simulink model "TV_2021"  (R2017b)
settings: Solver=VariableStepAuto  StartTime=0.0  StopTime=10.0  RelTol=1e-3
undefined symbols (not defined in the file): sigbuilder_block
libraries: simulink x6
(part 2 of 13)

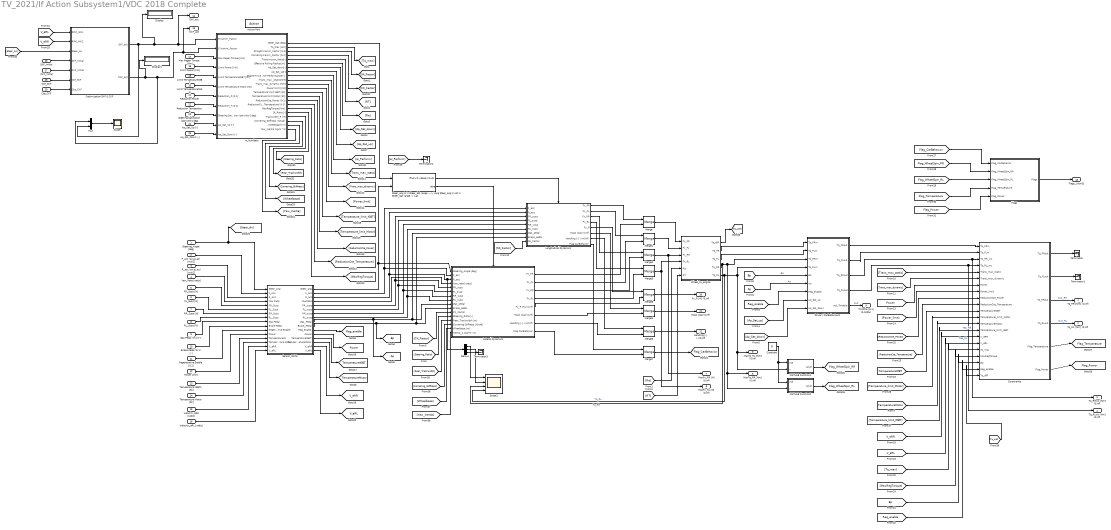
== system TV_2021/If Action Subsystem1/VDC 2018 Complete ==
  Steering_Angle [deg] : Inport
  F_acc (ax,ay,az) [m/s2] : Inport  Port=2
  R_acc (ax,ay,az) [m/s2] : Inport  Port=3
  Yaw_Rate [rad/s] : Inport  Port=4
  FR_Susp [N] : Inport  Port=5
  FL_Susp [N] : Inport  Port=6
  RR_Susp [N] : Inport  Port=7
  RL_Susp [N] : Inport  Port=8
  Gas Pedal (0-1) [-] : Inport  Port=9
  Brake Pedal (0-1) [-] : Inport  Port=10
  Regenerative Enable [0,1] : Inport  Port=11
  Power [kW] : Inport  Port=12
  Temperature IGBTs [ºC] : Inport  Port=13
  Temperature Motor [ºC] : Inport  Port=14
  Velocity_eRR [rad/s] : Inport  Port=15
  Velocity_eRL [rad/s] : Inport  Port=16
  Max Regen Torque [Nm] : Inport  Port=17
  Limit Power [kW] : Inport  Port=18
  Limit TemperatureIGBT : Inport  Port=19
  Limit TemperatureMotor : Inport  Port=20
  Reduction Power : Inport  Port=21
  Reduction Temperature : Inport  Port=22
  Steering Saturation (per site) [deg] : Inport  Port=23
  Ap_Sat_Up [-] : Inport  Port=24
  Ap_Sat_Down [-] : Inport  Port=25
  SKF_Initial : Inport  Port=26
  CKF_Initial : Inport  Port=27
  Cte_SKF : Inport  Port=28
  Cte_CKF : Inport  Port=29
  Action Port : ActionPort
  Constant : Constant  Value=0
  Constraints : Subsystem
  Demux : Demux  Outputs=3
  Display : Display
  Display1 : Display
  Driver / CarBehaviours : Subsystem
  Flags : Subsystem
  In_Numbers : Subsystem
  Lateral Dynamics : Subsystem  TreatAsAtomicUnit=on
  Longitudinal Dynamics : Subsystem  TreatAsAtomicUnit=on
  MATLAB Function1 : MATLAB Function  TreatAsAtomicUnit=on
  MATLAB Function2 : MATLAB Function  TreatAsAtomicUnit=on
  Merge{,1..7} (8 alike) : Merge
  Mux : Mux  Inputs=2
  Optimization SKF & CKF : Subsystem
  Scope : Scope
  Scope1 : Scope  NumInputPorts=4
  Sensor_DATA : Subsystem
  "Steer_ang is in Steer_Sat range ---> Long Steer_ang is not in Steer_Sat range -> Lat " : If  NumInputs=2  IfExpression=u2>=-u1&u2<=u1
  Terminator{,1..3} (4 alike) : Terminator
  Wheel_to_engine : Subsystem
  Tq_RR [Nm] (0,inf) : Outport
  Tq_RL [Nm] (0,inf) : Outport  Port=2
  Tq_RRwc [Nm] (0,inf) : Outport  Port=3
  Tq_RLwc [Nm] (0,inf) : Outport  Port=4
  MaxTq_RR [Nm] (0,inf) : Outport  Port=5
  MaxTq_RL [Nm] (0,inf) : Outport  Port=6
  MaxFx_RR [N] (0,inf) : Outport  Port=7
  MaxFx_RL [N] (0,inf) : Outport  Port=8
  Throttle [0-1] (0-100%) : Outport  Port=9
  Fy_R [N] (0,inf) : Outport  Port=10
  Mass [kg] (0,inf) : Outport  Port=11
  Handling [-] (-inf,inf) : Outport  Port=12
  Flags_[num5] : Outport  Port=13
  SKF_act : Outport  Port=14
  CKF_act : Outport  Port=15
  tag scope: Ap=global, Bp=global, Flag_CarBehavior=global, Flag_Power=global, Flag_Temperature=global, Flag_WheelSpin_RL=global, Flag_WheelSpin_RR=global, Power=global, Reg_enable=global, TemperatureIGBT=global, TemperatureMotor=global, V_eRL=global, V_eRR=global
  wires:
  "Steer_ang is in Steer_Sat range ---> Long Steer_ang is not in Steer_Sat range -> Lat "/1 -> Longitudinal Dynamics/Action
  "Steer_ang is in Steer_Sat range ---> Long Steer_ang is not in Steer_Sat range -> Lat "/2 -> Lateral Dynamics/Action
  Sensor_DATA/8(RL_susp) -> Longitudinal Dynamics/6(RL_susp), Lateral Dynamics/8(RL_susp)
  In_Numbers/3(Straight Kamm_Factor [0-2]) -> [SK_Factor]
  In_Numbers/1(Steer_Sat [deg]) -> "Steer_ang is in Steer_Sat range ---> Long Steer_ang is not in Steer_Sat range -> Lat "/1
  In_Numbers/2(Tq_Max [Nm]) -> [Tq_max]
  Sensor_DATA/9(Gas_Pedal) -> [Ap], Lateral Dynamics/9(Gas_pedal), Longitudinal Dynamics/7(Gas_pedal)
  In_Numbers/6(Effective Rolling Radius[m]) -> [Re]
  In_Numbers/5(Transmision_Ratio[-]) -> [RT]
  Sensor_DATA/7(RR_susp) -> Longitudinal Dynamics/5(RR_susp), Lateral Dynamics/7(RR_susp)
  In_Numbers/8(Ap_Sat_up[-]) -> [Ap_Sat_up]
  In_Numbers/7(Ap_Sat_down[-]) -> [Ap_Sat_down]
  Driver / CarBehaviours/3(Tq_RRout) -> Tq_RRwc [Nm] (0,inf)/1, Constraints/3(Tq_RR_wc)  "Teo_RR"
  Sensor_DATA/2(F_acc) -> Longitudinal Dynamics/1(F_acc), Lateral Dynamics/2(F_acc)
  Sensor_DATA/3(R_acc) -> Longitudinal Dynamics/2(R_acc), Demux/1, Lateral Dynamics/3(R_acc)
  Sensor_DATA/10(Brake_Pedal) -> [Bp], Lateral Dynamics/10(Brake_pedal), Longitudinal Dynamics/8(Brake_pedal)
  Sensor_DATA/6(FL_susp) -> Longitudinal Dynamics/4(FL_susp), Lateral Dynamics/6(FL_susp)
  Sensor_DATA/11(Reg_Enable) -> [Reg_enable]
  Sensor_DATA/5(FR_susp) -> Longitudinal Dynamics/3(FR_susp), Lateral Dynamics/5(FR_susp)
  Sensor_DATA/1(Steer_ang) -> Lateral Dynamics/1(Steering_Angle [deg]), "Steer_ang is in Steer_Sat range ---> Long Steer_ang is not in Steer_Sat range -> Lat "/2
  Wheel_to_engine/5(Tq_RL) -> Scope1/4, MaxTq_RL [Nm] (0,inf)/1, MATLAB Function1/2(v), Driver / CarBehaviours/4("Tq_RLin ")  "Tq_RL"
  [Trans_max_dynamic] -> Constraints/6(Trans_max_dynamic)
  [Power_limit] -> Constraints/8(Power_limit)
  In_Numbers/15(ReductionCte_Power (0-1)) -> [ReductionCte_Power]
  Driver / CarBehaviours/5(out_Throttle) -> Throttle [0-1] (0-100%)/1  "Out"
  Wheel_to_engine/4(Tq_RR) -> Scope1/3, MATLAB Function2/2(v), MaxTq_RR [Nm] (0,inf)/1, Driver / CarBehaviours/3(Tq_RRin)  "Tq_RR"
  Wheel_to_engine/3(Tq_FL) -> Driver / CarBehaviours/2(Tq_FLin)
  In_Numbers/11(Trans_max_dynamic [Nm]) -> [Trans_max_dynamic]
  [Reg_enable] -> Driver / CarBehaviours/7(Reg_enable)
  [ReductionCte_Power] -> Constraints/9(ReductionCte_Power)
  [Ap_Sat_up] -> Driver / CarBehaviours/8(Ap_Sat_up)
  In_Numbers/10(Trans_max _static[Nm]) -> [Trans_max_static]
  [Ap] -> Driver / CarBehaviours/6(Ap)  "Ap"
  [Power] -> Constraints/7(Power)
  In_Numbers/12("Power limit [KW] ") -> [Power_limit]
  [Ap_Sat_down] -> Driver / CarBehaviours/9(Ap_Sat_down)
  Driver / CarBehaviours/4(Tq_RLout) -> Tq_RLwc [Nm] (0,inf)/1, Constraints/4("Tq_RL_wc ")  "Teo_RL"
  Driver / CarBehaviours/2("Tq_FLout ") -> Constraints/2(Tq_FLin)
  Steering_Angle [deg]/1 -> [Steer_An], Sensor_DATA/1(Steer_Ang)
  Wheel_to_engine/2(Tq_FR) -> Driver / CarBehaviours/1(Tq_FRin)
  Driver / CarBehaviours/1(Tq_FRout) -> Constraints/1(Tq_FRin)
  [Trans_max_static] -> Constraints/5("Trans_max_static ")
  [Temperature_limit_IGBT] -> Constraints/14(Temperature_limit_IGBT)
  [Bp] -> Constraints/19(Bp)
  Sensor_DATA/16(V_eRL) -> [V_eRL]
  In_Numbers/17(MaxRegTorque [Nm]) -> [MaxRegTorque]
  [TemperatureIGBT] -> Constraints/11(TemperatureIGBT)
  [Reg_enable] -> Constraints/20(Reg_enable)
  In_Numbers/9(Engine+Inverter Performance[-]) -> [ei_Perform]
  [Bp] -> Driver / CarBehaviours/5(Bp)  "Bp"
  [Tq_max] -> Constraints/17(Tq_max)
  RR_Susp [N]/1 -> Sensor_DATA/7(RR_Susp)
  Power [kW]/1 -> Sensor_DATA/12("Power ")
  Sensor_DATA/12(Power) -> [Power]
  Sensor_DATA/15("V_eRR ") -> [V_eRR]
  [V_eRR] -> Constraints/15(V_eRR)
  Regenerative Enable [0,1]/1 -> Sensor_DATA/11(Regenerative Enable)
  Brake Pedal (0-1) [-]/1 -> Sensor_DATA/10(Brake Pedal)
  [V_eRL] -> Constraints/16(V_eRL)
  In_Numbers/13(Temperature limit IGBT [ºC]) -> [Temperature_limit_IGBT]
  FL_Susp [N]/1 -> Sensor_DATA/6(FL_Susp)
  FR_Susp [N]/1 -> Sensor_DATA/5(FR_Susp)
  R_acc (ax,ay,az) [m/s2]/1 -> Sensor_DATA/3(R_Acc)
  F_acc (ax,ay,az) [m/s2]/1 -> Sensor_DATA/2("F_Acc ")
  RL_Susp [N]/1 -> Sensor_DATA/8(RL_Susp)
  Gas Pedal (0-1) [-]/1 -> Sensor_DATA/9(Gas Pedal)
  Temperature IGBTs [ºC]/1 -> Sensor_DATA/13(TemperatureIN)
  Velocity_eRR [rad/s]/1 -> Sensor_DATA/15(V_eRR)
  Velocity_eRL [rad/s]/1 -> Sensor_DATA/16("V_eRL ")
  Constraints/1(Tq_FRout) -> Terminator/1
  Constraints/2("Tq_FLout ") -> Terminator1/1
  In_Numbers/4(Cornering Kamm_Factor [0-2]) -> [CK_Factor]
  [Re] -> Wheel_to_engine/5(Re)
  [RT] -> Wheel_to_engine/6(RT)
  Merge3/1 -> MaxFx_RL [N] (0,inf)/1, Wheel_to_engine/4("Fx_RL ")
  Merge2/1 -> Wheel_to_engine/3("Fx_RR "), MaxFx_RR [N] (0,inf)/1
  Merge1/1 -> Wheel_to_engine/2("Fx_FL ")
  Max Regen Torque [Nm]/1 -> In_Numbers/3(Max Regen Torque [Nm])
  Limit Power [kW]/1 -> In_Numbers/4(Limit Power [kW])
  Limit TemperatureIGBT/1 -> In_Numbers/5(Limit TemperatureIGBT [ºC])
  Reduction Power/1 -> In_Numbers/7(Reduction_P [0-1])
  [CK_Factor] -> Lateral Dynamics/11(CK_Factor)
  [SK_Factor] -> Longitudinal Dynamics/9(SK_Factor)
  Longitudinal Dynamics/1(Fx_FR) -> Merge/1
  Longitudinal Dynamics/2(Fx_FL) -> Merge1/1
  Longitudinal Dynamics/3("Fx_RR ") -> Merge2/1
  Longitudinal Dynamics/4("Fx_RL ") -> Merge3/1
  Lateral Dynamics/1(Fx_FR) -> Merge/2
  Lateral Dynamics/2(Fx_FL) -> Merge1/2
  Lateral Dynamics/3("Fx_RR ") -> Merge2/2
  Lateral Dynamics/4("Fx_RL ") -> Merge3/2
  Merge/1 -> Wheel_to_engine/1("Fx_FR ")
  Steering Saturation (per site) [deg]/1 -> In_Numbers/9(Steering Saturation (per site) [deg])
  Ap_Sat_Up [-]/1 -> In_Numbers/10(Ap_Sat_Up [-])
  Ap_Sat_Down [-]/1 -> In_Numbers/11(Ap_Sat_Down [-])
  [MaxRegTorque] -> Constraints/18(MaxRegTorque)
  [ei_Perform] -> Terminator2/1
  Merge4/1 -> Mass [kg] (0,inf)/1
  Longitudinal Dynamics/6(Mass [kg] (0,inf)) -> Merge4/1
  Lateral Dynamics/6(" Mass [kg] (0,inf)") -> Merge4/2
  Longitudinal Dynamics/7(Handling [-] (-inf,inf)) -> Merge5/1
  Lateral Dynamics/7(Handling [-] (-inf,inf)) -> Merge5/2
  Merge5/1 -> Handling [-] (-inf,inf)/1
  Merge6/1 -> Fy_R [N] (0,inf)/1
  Lateral Dynamics/5(Fy_R [N] (0,inf)) -> Merge6/2
  Longitudinal Dynamics/5(Fy_R) -> Merge6/1
  In_Numbers/16(ReductionCte_Temperature (0-1)) -> [ReductionCte_Temperature]
  Reduction Temperature/1 -> In_Numbers/8(Reduction_T [0-1])
  [ReductionCte_Temperature] -> Constraints/10(ReductionCte_Temperature)
  Constraints/3(Tq_RRout) -> Tq_RR [Nm] (0,inf)/1  "Out_RR"
  Constraints/4(Tq_RLout) -> Tq_RL [Nm] (0,inf)/1  "Out_RL"
  Temperature Motor [ºC]/1 -> Sensor_DATA/14(Temperature Motor)
  Sensor_DATA/13(TemperatureIGBT) -> [TemperatureIGBT]
  Sensor_DATA/14(TemperatureMotor) -> [TemperatureMotor]
  [TemperatureMotor] -> Constraints/13(TemperatureIMotor)
  [Temperature_limit_Motor] -> Constraints/12(TemperatureI_limit_Motor)
  In_Numbers/14(Temperature limit Motor [ºC]) -> [Temperature_limit_Motor]
  Limit TemperatureMotor/1 -> In_Numbers/6(Limit Temperature Motor [ºC])
  Merge7/1 -> [Flag_CarBehavior]
  Longitudinal Dynamics/8(Flag CarBehavior) -> Merge7/1
  Lateral Dynamics/8(Flag CarBehavior) -> Merge7/2
  MATLAB Function2/1(value) -> [Flag_WheelSpin_RL]
  MATLAB Function1/1(value) -> [Flag_WheelSpin_RR]
  Constant/1 -> MATLAB Function2/1(cte), MATLAB Function1/1(cte)
  Constraints/5(Flag_Temperature) -> [Flag_Temperature]
  Constraints/6(Flag_Power) -> [Flag_Power]
  Flags/1(Flags) -> Flags_[num5]/1
  [Flag_WheelSpin_RL] -> Flags/3(Flag_WheelSpin_RL)
  [Flag_WheelSpin_RR] -> Flags/2(Flag_WheelSpin_RR)
  [Flag_CarBehavior] -> Flags/1(Flag_CarBehavior)
  [Flag_Temperature] -> Flags/4(Flag_Temperature)
  [Flag_Power] -> Flags/5(Flag_Power)
  Optimization SKF & CKF/1(SKF_act) -> In_Numbers/1(S-Kamm_Factor), SKF_act/1, Display/1, Mux/2
  CKF_Initial/1 -> Optimization SKF & CKF/5(CKF_Initial)
  [Steer_An] -> Optimization SKF & CKF/3(Steer_An)
  [V_eRR] -> Optimization SKF & CKF/2(RPM_INV2)
  Cte_SKF/1 -> Optimization SKF & CKF/6(Cte_SKF)
  Cte_CKF/1 -> Optimization SKF & CKF/7(Cte_CKF)
  SKF_Initial/1 -> Optimization SKF & CKF/4(SKF_Initial)
  [V_eRL] -> Optimization SKF & CKF/1(RPM_INV1)
  Optimization SKF & CKF/2(CKF_act) -> Display1/1, Mux/1, In_Numbers/2(C-Kamm_Factor), CKF_act/1
  Mux/1 -> Scope/1
  Yaw_Rate [rad/s]/1 -> Sensor_DATA/4(Yaw Rate)
  Sensor_DATA/4(YawRate) -> Lateral Dynamics/4(Yaw_rate [rad/s])
  In_Numbers/18(St_Ratio [-]) -> [Steering_Ratio]
  [Steering_Ratio] -> Lateral Dynamics/12(Steering_Ratio [-])
  Demux/2 -> Scope1/2
  Demux/1 -> Scope1/1
  Demux/3 -> Terminator3/1
  In_Numbers/19(Trackwidth_R (m)) -> [Rear_Trackwidth]
  In_Numbers/20(Cornering_Stiffness (N/rad)) -> [Cornering_Stiffness]
  In_Numbers/21(Wheelbase (m)) -> [Wheelbase]
  [Rear_Trackwidth] -> Lateral Dynamics/13(Rear_Trackwidth [m])
  [Cornering_Stiffness] -> Lateral Dynamics/14(Cornering Stiffness [N/rad])
  [Wheelbase] -> Lateral Dynamics/15(Wheelbase [m])
  In_Numbers/22(Yaw_Inertia (kg/m^3)) -> [Yaw_Inertia]
  [Yaw_Inertia] -> Lateral Dynamics/16(Inertia_Z [kg*m^2])
  Wheel_to_engine/1(Tq_diff) -> [Tq_diff]
  [Tq_diff] -> Constraints/21(Tq_diff)

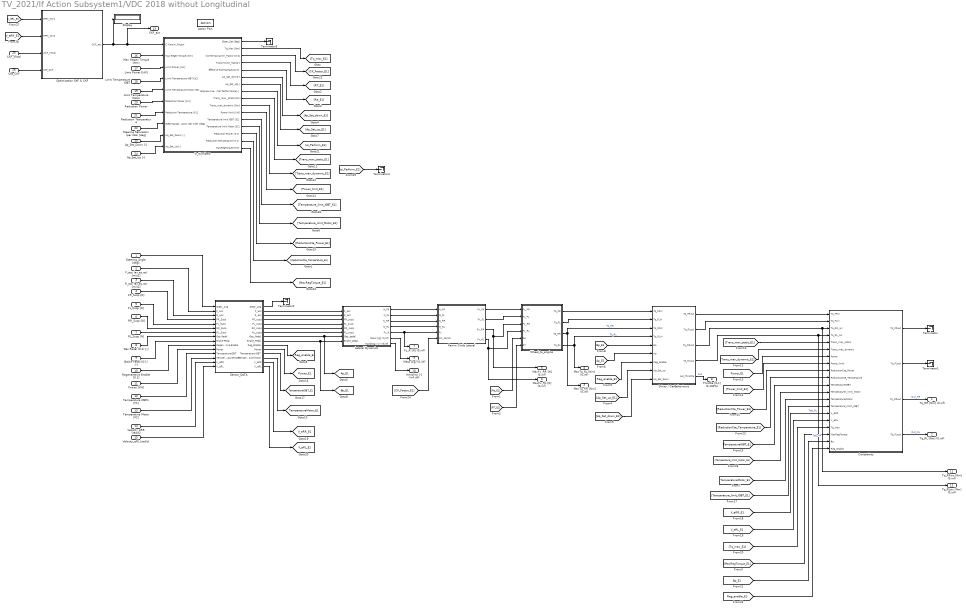
== system TV_2021/If Action Subsystem1/VDC 2018 without Longitudinal ==
  Steering_Angle [deg] : Inport
  F_acc (ax,ay,az) [m/s2] : Inport  Port=2
  R_acc (ax,ay,az) [m/s2] : Inport  Port=3
  FR_Susp [N] : Inport  Port=4
  FL_Susp [N] : Inport  Port=5
  RR_Susp [N] : Inport  Port=6
  RL_Susp [N] : Inport  Port=7
  Gas Pedal (0-1) [-] : Inport  Port=8
  Brake Pedal (0-1) [-] : Inport  Port=9
  Regenerative Enable [0,1] : Inport  Port=10
  Power [kW] : Inport  Port=11
  Temperature IGBTs [ºC] : Inport  Port=12
  Temperature Motor [ºC] : Inport  Port=13
  Velocity_eRR [rad/s] : Inport  Port=14
  Velocity_eRL [rad/s] : Inport  Port=15
  Max Regen Torque [Nm] : Inport  Port=16
  Limit Power [kW] : Inport  Port=17
  Limit Temperature IGBT : Inport  Port=18
  Limit Temperature Motor : Inport  Port=19
  Reduction Power : Inport  Port=20
  Reduction Temperature : Inport  Port=21
  Steering Saturation (per site) [deg] : Inport  Port=22
  Ap_Sat_Down [-] : Inport  Port=23
  Ap_Sat_Up [-] : Inport  Port=24
  CKF_Initial : Inport  Port=25
  Cte_CKF : Inport  Port=26
  Action Port : ActionPort
  Constraints : Subsystem
  Display : Display
  Driver / CarBehaviours : Subsystem
  In_Numbers : Subsystem
  Kamm Circle Lateral : Subsystem
  Lateral Dynamics : Subsystem
  Optimization SKF & CKF : Subsystem
  Sensor_DATA : Subsystem
  Terminator{,1..2,4..5} (5 alike) : Terminator
  Wheel_to_engine : Subsystem
  Tq_RR [Nm] (0,inf) : Outport
  Tq_RL [Nm] (0,inf) : Outport  Port=2
  MaxTq_RR [Nm] (0,inf) : Outport  Port=3
  MaxTq_RL [Nm] (0,inf) : Outport  Port=4
  MaxFx_RR [N] (0,inf) : Outport  Port=5
  MaxFx_RL [N] (0,inf) : Outport  Port=6
  Fy_R [N] (0,inf) : Outport  Port=7
  Throttle [0-1] (0-100%) : Outport  Port=8
  Mass [kg] (0,inf) : Outport  Port=9
  Handling [-] (-inf,inf) : Outport  Port=10
  Tq_RRwc [Nm] (0,inf) : Outport  Port=11
  Tq_RLwc [Nm] (0,inf) : Outport  Port=12
  CKF_act : Outport  Port=13
  tag scope: Ap_E1=global, Bp_E1=global, Power_E1=global, Reg_enable_E1=global, TemperatureIGBT_E1=global, TemperatureMotor_E1=global, V_eRL_E1=global, V_eRR_E1=global
  wires:
  Sensor_DATA/7(RL_susp) -> Lateral Dynamics/6(RL_susp)
  In_Numbers/2(Tq_Max [Nm]) -> [Tq_max_E1]
  Sensor_DATA/8(Gas_Pedal) -> [Ap_E1], Lateral Dynamics/7(Gas_pedal)
  In_Numbers/5(Effective Rolling Radius[m]) -> [Re_E1]
  In_Numbers/4(Transmision_Ratio[-]) -> [RT_E1]
  Sensor_DATA/6(RR_susp) -> Lateral Dynamics/5(RR_susp)
  In_Numbers/7(Ap_Sat_up[-]) -> [Ap_Sat_up_E1]
  In_Numbers/6(Ap_Sat_down[-]) -> [Ap_Sat_down_E1]
  Sensor_DATA/2(F_acc) -> Lateral Dynamics/1(F_acc)
  Sensor_DATA/3(R_acc) -> Lateral Dynamics/2(R_acc)
  Sensor_DATA/9(Brake_Pedal) -> [Bp_E1], Lateral Dynamics/8(Brake_pedal)
  Sensor_DATA/5(FL_susp) -> Lateral Dynamics/4(FL_susp)
  Sensor_DATA/10(Reg_Enable) -> [Reg_enable_E1]
  Sensor_DATA/4(FR_susp) -> Lateral Dynamics/3(FR_susp)
  Wheel_to_engine/4(Tq_RL) -> MaxTq_RL [Nm] (0,inf)/1, Driver / CarBehaviours/4("Tq_RLin ")  "Tq_RL"
  In_Numbers/14(Reduction Power (0-1)) -> [ReductionCte_Power_E1]
  Wheel_to_engine/3(Tq_RR) -> MaxTq_RR [Nm] (0,inf)/1, Driver / CarBehaviours/3(Tq_RRin)  "Tq_RR"
  Wheel_to_engine/2(Tq_FL) -> Driver / CarBehaviours/2(Tq_FLin)
  In_Numbers/10(Trans_max_dynamic [Nm]) -> [Trans_max_dynamic_E1]
  [Reg_enable_E1] -> Driver / CarBehaviours/7(Reg_enable)
  [Ap_Sat_up_E1] -> Driver / CarBehaviours/8(Ap_Sat_up)
  In_Numbers/9(Trans_max _static[Nm]) -> [Trans_max_static_E1]
  [Ap_E1] -> Driver / CarBehaviours/6(Ap)
  In_Numbers/11("Power limit [KW] ") -> [Power_limit_E1]
  [Ap_Sat_down_E1] -> Driver / CarBehaviours/9(Ap_Sat_down)
  Steering_Angle [deg]/1 -> Sensor_DATA/1(Steer_Ang)
  Wheel_to_engine/1(Tq_FR) -> Driver / CarBehaviours/1(Tq_FRin)
  Sensor_DATA/15(V_eRL) -> [V_eRL_E1]
  In_Numbers/16(MaxRegTorque [Nm]) -> [MaxRegTorque_E1]
  In_Numbers/8(Engine+Inverter Performance[-]) -> [ei_Perform_E1]
  [Bp_E1] -> Driver / CarBehaviours/5(Bp)
  Sensor_DATA/12(Temperature IGBT) -> [TemperatureIGBT_E1]
  RR_Susp [N]/1 -> Sensor_DATA/6(RR_Susp)
  Power [kW]/1 -> Sensor_DATA/11("Power ")
  Sensor_DATA/11(Power) -> [Power_E1]
  Sensor_DATA/14("V_eRR ") -> [V_eRR_E1]
  Regenerative Enable [0,1]/1 -> Sensor_DATA/10(Regenerative Enable)
  Brake Pedal (0-1) [-]/1 -> Sensor_DATA/9(Brake Pedal)
  In_Numbers/12(Temperature limit IGBT [ºC]) -> [Temperature_limit_IGBT_E1]
  FL_Susp [N]/1 -> Sensor_DATA/5(FL_Susp)
  FR_Susp [N]/1 -> Sensor_DATA/4(FR_Susp)
  R_acc (ax,ay,az) [m/s2]/1 -> Sensor_DATA/3(R_Acc)
  F_acc (ax,ay,az) [m/s2]/1 -> Sensor_DATA/2("F_Acc ")
  RL_Susp [N]/1 -> Sensor_DATA/7(RL_Susp)
  Gas Pedal (0-1) [-]/1 -> Sensor_DATA/8(Gas Pedal)
  Temperature IGBTs [ºC]/1 -> Sensor_DATA/12(TemperatureIGBT)
  Velocity_eRR [rad/s]/1 -> Sensor_DATA/14(V_eRR)
  Velocity_eRL [rad/s]/1 -> Sensor_DATA/15("V_eRL ")
  Max Regen Torque [Nm]/1 -> In_Numbers/2(Max Regen Torque [Nm])
  Limit Power [kW]/1 -> In_Numbers/3(Limit Power [kW])
  Limit Temperature IGBT/1 -> In_Numbers/4(Limit Temperature IGBT [ºC])
  Reduction Power/1 -> In_Numbers/6(Reduction Power [0-1])
  In_Numbers/3(Cornering Kamm_Factor [0-2]) -> [CK_Factor_E1]
  [Re_E1] -> Wheel_to_engine/5(Re)
  [RT_E1] -> Wheel_to_engine/6(RT)
  Ap_Sat_Up [-]/1 -> In_Numbers/10(Ap_Sat_Up [-])
  Ap_Sat_Down [-]/1 -> In_Numbers/9(Ap_Sat_Down [-])
  Steering Saturation (per site) [deg]/1 -> In_Numbers/8(Steering Saturation (per site) [deg])
  [CK_Factor_E1] -> Kamm Circle Lateral/6(CK_Factor)
  Kamm Circle Lateral/1(Fx_FR) -> Wheel_to_engine/1("Fx_FR ")
  Kamm Circle Lateral/2(Fx_FL) -> Wheel_to_engine/2("Fx_FL ")
  Kamm Circle Lateral/3("Fx_RR ") -> MaxFx_RR [N] (0,inf)/1, Wheel_to_engine/3("Fx_RR ")
  Kamm Circle Lateral/4("Fx_RL ") -> MaxFx_RL [N] (0,inf)/1, Wheel_to_engine/4("Fx_RL ")
  Sensor_DATA/1(Steer_ang) -> Terminator2/1
  Lateral Dynamics/1(N_FR) -> Kamm Circle Lateral/1("N_FR ")
  Lateral Dynamics/2("N_FL ") -> Kamm Circle Lateral/2(N_FL)
  Lateral Dynamics/3("N_RR ") -> Kamm Circle Lateral/3(N_RR)
  Lateral Dynamics/4(N_RL) -> Kamm Circle Lateral/4(N_RL)
  Lateral Dynamics/5(Fy_R) -> Fy_R [N] (0,inf)/1, Kamm Circle Lateral/5(Fy)
  Driver / CarBehaviours/5(out_Throttle) -> Throttle [0-1] (0-100%)/1  "Out"
  [ei_Perform_E1] -> Terminator4/1
  In_Numbers/1(Steer_Sat [deg]) -> Terminator5/1
  Lateral Dynamics/6(Mass [kg] (0,inf)) -> Mass [kg] (0,inf)/1
  Lateral Dynamics/7(Handling [-] (-inf,inf)) -> Handling [-] (-inf,inf)/1
  In_Numbers/15(Reduction Temperature (0-1)) -> [ReductionCte_Temperature_E1]
  Reduction Temperature/1 -> In_Numbers/7(Reduction Temperature [0-1])
  Driver / CarBehaviours/3(Tq_RRout) -> Tq_RRwc [Nm] (0,inf)/1, Constraints/3(Tq_RR_wc)  "Teo_RR"
  [Trans_max_dynamic_E1] -> Constraints/6(Trans_max_dynamic)
  [Power_limit_E1] -> Constraints/8(Power_limit)
  [ReductionCte_Power_E1] -> Constraints/9(ReductionCte_Power)
  [Power_E1] -> Constraints/7(Power)
  Driver / CarBehaviours/4(Tq_RLout) -> Tq_RLwc [Nm] (0,inf)/1, Constraints/4("Tq_RL_wc ")  "Teo_RL"
  Driver / CarBehaviours/2("Tq_FLout ") -> Constraints/2(Tq_FLin)
  Driver / CarBehaviours/1(Tq_FRout) -> Constraints/1(Tq_FRin)
  [Trans_max_static_E1] -> Constraints/5("Trans_max_static ")
  [Temperature_limit_IGBT_E1] -> Constraints/14(Temperature_limit_IGBT)
  [Bp_E1] -> Constraints/19(Bp)
  [TemperatureIGBT_E1] -> Constraints/11(TemperatureIGBT)
  [Reg_enable_E1] -> Constraints/20(Reg_enable)
  [Tq_max_E1] -> Constraints/17(Tq_max)
  [V_eRR_E1] -> Constraints/15(V_eRR)
  [V_eRL_E1] -> Constraints/16(V_eRL)
  Constraints/1(Tq_FRout) -> Terminator/1
  Constraints/2("Tq_FLout ") -> Terminator1/1
  [MaxRegTorque_E1] -> Constraints/18(MaxRegTorque)
  [ReductionCte_Temperature_E1] -> Constraints/10(ReductionCte_Temperature)
  Constraints/3(Tq_RRout) -> Tq_RR [Nm] (0,inf)/1  "Out_RR"
  Constraints/4(Tq_RLout) -> Tq_RL [Nm] (0,inf)/1  "Out_RL"
  [TemperatureMotor_E1] -> Constraints/13(TemperatureIMotor)
  [Temperature_limit_Motor_E1] -> Constraints/12(TemperatureI_limit_Motor)
  Limit Temperature Motor/1 -> In_Numbers/5(Limit Temperature Motor [ºC])
  In_Numbers/13(Temperature limit Motor [ºC]) -> [Temperature_limit_Motor_E1]
  Temperature Motor [ºC]/1 -> Sensor_DATA/13(TemperatureMotor)
  Sensor_DATA/13(Temperature Motor) -> [TemperatureMotor_E1]
  [V_eRR_E1] -> Optimization SKF & CKF/2(RPM_INV2)
  CKF_Initial/1 -> Optimization SKF & CKF/3(CKF_Initial)
  Cte_CKF/1 -> Optimization SKF & CKF/4(Cte_CKF)
  Optimization SKF & CKF/1(CKF_act) -> Display/1, In_Numbers/1(C-Kamm_Factor), CKF_act/1
  [V_eRL_E1] -> Optimization SKF & CKF/1(RPM_INV1)

== system TV_2021/Vehicle Dynamics Control 1/Rigid Axle ==
  "Ap_Sat_up " : Inport
  Ap_Sat_down : Inport  Port=2
  Gas Pedal [0-1] : Inport  Port=3
  Action Port : ActionPort
  Accelerating : Subsystem
  Torque_RL [Nm] : Constant  Value=60
  Torque_RR [Nm] : Constant  Value=60
  Tq_RR_E3 : Outport
  Tq_RL_E3 : Outport  Port=2
  wires:
  Ap_Sat_down/1 -> Accelerating/3(Ap_Sat_down)
  "Ap_Sat_up "/1 -> Accelerating/2("Ap_Sat_up ")
  Gas Pedal [0-1]/1 -> Accelerating/1(Ap)
  Accelerating/1("Tq_RR ") -> Tq_RR_E3/1
  Accelerating/2(Tq_RL) -> Tq_RL_E3/1
  Torque_RL [Nm]/1 -> Accelerating/5("Tq_RL ")
  Torque_RR [Nm]/1 -> Accelerating/4(Tq_RR)

== system TV_2021/Vehicle Dynamics Control 1/Steering TV 2017 with TC ==
  "Ap_Sat_up " : Inport
  Ap_Sat_down : Inport  Port=2
  Gas Pedal [0-1] : Inport  Port=3
  Steering_Angle [deg] : Inport  Port=4
  "Steering Wheel Saturation (per site) " : Inport  Port=5
  Power : Inport  Port=6
  Temperature_limit_IGBT : Inport  Port=7
  TemperatureIGBT : Inport  Port=8
  Temperature_limit_Motor : Inport  Port=9
  TemperatureMotor : Inport  Port=10
  Reduction_Power : Inport  Port=11
  Reduction_Temperature : Inport  Port=12
  SKF_Initial : Inport  Port=13
  CKF_Initial : Inport  Port=14
  Cte_SKF : Inport  Port=15
  Cte_CKF : Inport  Port=16
  Vel_eRL : Inport  Port=17
  Vel_eRR : Inport  Port=18
  Temp_Celdas : Inport  Port=19
  Lim_Temp_Celdas : Inport  Port=20
  Voltage : Inport  Port=21
  Corriente : Inport  Port=22
  Action Port : ActionPort
  Accelerating : Subsystem
  CKF : Display
  Constraints : Subsystem
  Display{2..6} (5 alike) : Display
  If : If  NumInputs=2  IfExpression=-u2 <= u1 & u1 <= u2
  Lateral Dynamics : Subsystem  TreatAsAtomicUnit=on
  Longitudinal Dynamics : Subsystem  TreatAsAtomicUnit=on
  MATLAB Function1 : MATLAB Function  TreatAsAtomicUnit=on
  Merge : Merge
  Merge1 : Merge
  Mux : Mux  Inputs=2
  Optimization SKF & CKF : Subsystem
  SKF : Display
  Scope : Scope
  Steering TV 2017 without TC : MATLAB Function  TreatAsAtomicUnit=on
  Steering Wheel Maximum Angle : Constant  Value=140
  Tq_diff_max [Nm] : Constant  Value=100
  Tq_max [Nm] : Constant  Value=130
  Tq_RR_E2 : Outport
  Tq_RL_E2 : Outport  Port=2
  SKF_act : Outport  Port=3
  CKF_act : Outport  Port=4
  wires:
  Corriente/1 -> Constraints/13(Corriente)
  Voltage/1 -> Constraints/12(Voltage)
  Lim_Temp_Celdas/1 -> Constraints/7(Lim_Temp_Celdas)
  Temp_Celdas/1 -> Constraints/6(Temp_Celdas)
  Merge1/1 -> Accelerating/5("Tq_RL ")
  Merge/1 -> Accelerating/4(Tq_RR)
  Lateral Dynamics/1(Tq_RR_with_CKF) -> Merge/2
  Longitudinal Dynamics/1(Tq_RR_with_SKF) -> Merge/1
  Longitudinal Dynamics/2(Tq_RL_with_SKF) -> Merge1/1
  If/2 -> Lateral Dynamics/Action
  Lateral Dynamics/2(Tq_RL_with_CKF) -> Merge1/2
  If/1 -> Longitudinal Dynamics/Action
  Cte_CKF/1 -> Optimization SKF & CKF/7(Cte_CKF)
  CKF_Initial/1 -> Optimization SKF & CKF/5(CKF_Initial)
  Steering_Angle [deg]/1 -> Optimization SKF & CKF/3(Steer_An), MATLAB Function1/1(v)
  Optimization SKF & CKF/1(SKF_act) -> Mux/2, SKF/1, Longitudinal Dynamics/1(SKF), SKF_act/1
  Vel_eRR/1 -> Optimization SKF & CKF/2(RPM_INV2)
  Vel_eRL/1 -> Optimization SKF & CKF/1(RPM_INV1)
  Cte_SKF/1 -> Optimization SKF & CKF/6(Cte_SKF)
  Mux/1 -> Scope/1
  SKF_Initial/1 -> Optimization SKF & CKF/4(SKF_Initial)
  Optimization SKF & CKF/2(CKF_act) -> CKF_act/1, Lateral Dynamics/1(CKF), Mux/1, CKF/1
  TemperatureMotor/1 -> Constraints/5(Temperature_Motor)
  Temperature_limit_Motor/1 -> Constraints/4(Temperature_limit_Motor)
  MATLAB Function1/1(value) -> If/1, Steering TV 2017 without TC/1(sw_angle), Display4/1
  Accelerating/1("Tq_RR ") -> Constraints/8(Tq_RR), Display2/1
  Accelerating/2(Tq_RL) -> Constraints/9(Tq_RL), Display3/1
  Constraints/2(TQ_RL) -> Tq_RL_E2/1
  Constraints/1(TQ_RR) -> Tq_RR_E2/1
  Reduction_Power/1 -> Constraints/11(ReductionCte_Power)
  Reduction_Temperature/1 -> Constraints/10(ReductionCte_Temperature)
  TemperatureIGBT/1 -> Constraints/3(Temperature_IGBT)
  Temperature_limit_IGBT/1 -> Constraints/2(Temperature_limit_IGBT)
  Power/1 -> Constraints/1(Power)
  Steering TV 2017 without TC/2(tq_RL) -> Display6/1, Lateral Dynamics/3(Tq_RL), Longitudinal Dynamics/3(Tq_RL)
  Steering TV 2017 without TC/1(tq_RR) -> Lateral Dynamics/2(Tq_RR), Longitudinal Dynamics/2(Tq_RR), Display5/1
  "Steering Wheel Saturation (per site) "/1 -> Steering TV 2017 without TC/2(sw_saturation), If/2
  Steering Wheel Maximum Angle/1 -> MATLAB Function1/2(cte), Steering TV 2017 without TC/3(sw_max_angle)
  Tq_diff_max [Nm]/1 -> Steering TV 2017 without TC/5(tq_max_diff)
  Tq_max [Nm]/1 -> Steering TV 2017 without TC/4(tq_max)
  Ap_Sat_down/1 -> Accelerating/3(Ap_Sat_down)
  "Ap_Sat_up "/1 -> Accelerating/2("Ap_Sat_up ")
  Gas Pedal [0-1]/1 -> Accelerating/1(Ap)

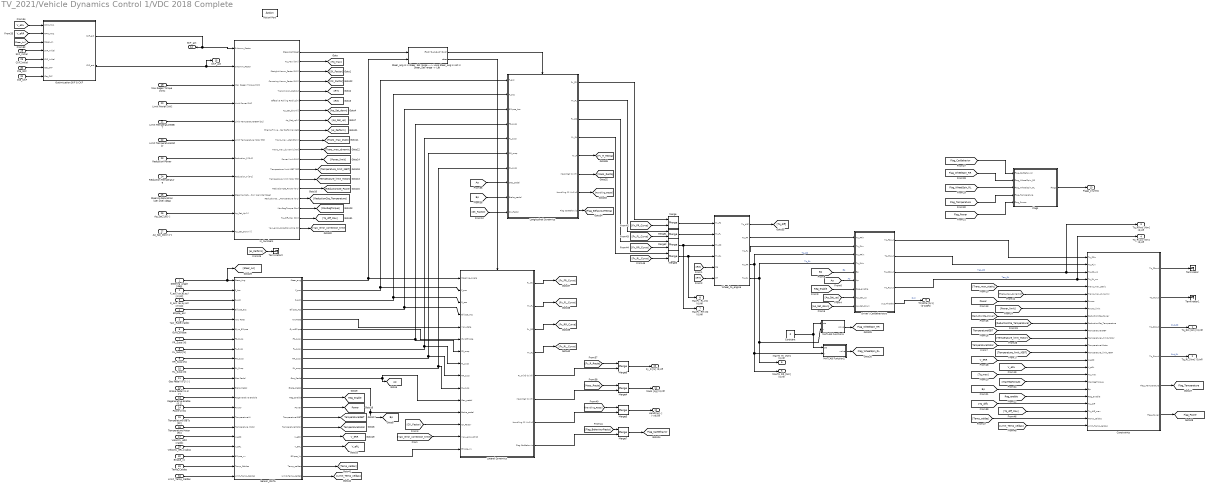
== system TV_2021/Vehicle Dynamics Control 1/VDC 2018 Complete ==
  Steering_Angle [deg] : Inport
  F_acc (ax,ay,az) [m/s2] : Inport  Port=2
  R_acc (ax,ay,az) [m/s2] : Inport  Port=3
  Ellipse_acc : Inport  Port=4
  Yaw_Rate [rad/s] : Inport  Port=5
  Gyro_Ellipse : Inport  Port=6
  FR_Susp [N] : Inport  Port=7
  FL_Susp [N] : Inport  Port=8
  RR_Susp [N] : Inport  Port=9
  RL_Susp [N] : Inport  Port=10
  Gas Pedal (0-1) [-] : Inport  Port=11
  Brake Pedal (0-1) [-] : Inport  Port=12
  Regenerative Enable [0,1] : Inport  Port=13
  Power [kW] : Inport  Port=14
  Temperature IGBTs [ºC] : Inport  Port=15
  Temperature Motor [ºC] : Inport  Port=16
  Velocity_eRR [rad/s] : Inport  Port=17
  Velocity_eRL [rad/s] : Inport  Port=18
  Max Regen Torque [Nm] : Inport  Port=19
  Limit Power [kW] : Inport  Port=20
  Limit TemperatureIGBT : Inport  Port=21
  Limit TemperatureMotor : Inport  Port=22
  Reduction Power : Inport  Port=23
  Reduction Temperature : Inport  Port=24
  Steering Saturation (per site) [deg] : Inport  Port=25
  Ap_Sat_Up [-] : Inport  Port=26
  Ap_Sat_Down [-] : Inport  Port=27
  SKF_Initial : Inport  Port=28
  CKF_Initial : Inport  Port=29
  Cte_SKF : Inport  Port=30
  Cte_CKF : Inport  Port=31
  Ellipse_vx : Inport  Port=32
  Temp_Celdas : Inport  Port=33
  Limit_Temp_Celdas : Inport  Port=34
  Action Port : ActionPort
  Constant : Constant  Value=0
  Constraints : Subsystem
  Driver / CarBehaviours : Subsystem
  Flags : Subsystem
  In_Numbers : Subsystem
  Lateral Dynamics : Subsystem  TreatAsAtomicUnit=on
  Longitudinal Dynamics : Subsystem  TreatAsAtomicUnit=on
  MATLAB Function1 : MATLAB Function  TreatAsAtomicUnit=on
  MATLAB Function2 : MATLAB Function  TreatAsAtomicUnit=on
  Merge{,1..7} (8 alike) : Merge
  Optimization SKF & CKF : Subsystem
  Sensor_DATA : Subsystem
  "Steer_ang is in Steer_Sat range ---> Long Steer_ang is not in Steer_Sat range -> Lat " : If  NumInputs=2  IfExpression=u2>=-u1&u2<=u1
  Terminator : Terminator
  Terminator1 : Terminator
  Terminator2 : Terminator
  Wheel_to_engine : Subsystem
  Tq_RR [Nm] (0,inf) : Outport
  Tq_RL [Nm] (0,inf) : Outport  Port=2
  Tq_RRwc [Nm] (0,inf) : Outport  Port=3
  Tq_RLwc [Nm] (0,inf) : Outport  Port=4
  MaxTq_RR [Nm] (0,inf) : Outport  Port=5
  MaxTq_RL [Nm] (0,inf) : Outport  Port=6
  MaxFx_RR [N] (0,inf) : Outport  Port=7
  MaxFx_RL [N] (0,inf) : Outport  Port=8
  Throttle [0-1] (0-100%) : Outport  Port=9
  Fy_R [N] (0,inf) : Outport  Port=10
  Mass [kg] (0,inf) : Outport  Port=11
  Handling [-] (-inf,inf) : Outport  Port=12
  Flags_[num5] : Outport  Port=13
  SKF_act : Outport  Port=14
  CKF_act : Outport  Port=15
  tag scope: Ap=global, Bp=global, Flag_CarBehavior=global, Flag_Power=global, Flag_Temperature=global, Flag_WheelSpin_RL=global, Flag_WheelSpin_RR=global, Power=global, Reg_enable=global, TemperatureIGBT=global, TemperatureMotor=global, V_eRL=global, V_eRR=global
  wires:
  [Limit_Temp_celdas] -> Constraints/24(Limit_Temp_celdas)
  [Temp_celdas] -> Constraints/23(Temp_celdas)
  Sensor_DATA/21(Limit_Temp_celdas) -> [Limit_Temp_celdas]
  Sensor_DATA/20(Temp_celdas) -> [Temp_celdas]
  Limit_Temp_Celdas/1 -> Sensor_DATA/21(Limit_Temp_Celdas)
  Temp_Celdas/1 -> Sensor_DATA/20(Temp_Celdas)
  [Tq_diff_Max] -> Constraints/22(Tq_diff_max)
  Sensor_DATA/19(Ellipse_Vx) -> Lateral Dynamics/15(Ellipse_Vx)
  Ellipse_vx/1 -> Sensor_DATA/19(Ellipse_vx)
  [Fx_RL_Curva] -> Merge3/2
  [Fx_RR_Curva] -> Merge2/2
  [Fx_FL_Curva] -> Merge1/2
  [Fx_FR_Curva] -> Merge/2
  Lateral Dynamics/4("Fx_RL ") -> [Fx_RL_Curva]
  Lateral Dynamics/3("Fx_RR ") -> [Fx_RR_Curva]
  Lateral Dynamics/2(Fx_FL) -> [Fx_FL_Curva]
  Lateral Dynamics/1(Fx_FR) -> [Fx_FR_Curva]
  [Flag_BehaviourRecta] -> Merge7/1
  [Handling_Recta] -> Merge5/1
  [Mass_Recta] -> Merge4/1
  [Fy_R_Recta] -> Merge6/1
  Longitudinal Dynamics/5(Fy_R) -> [Fy_R_Recta]
  Longitudinal Dynamics/8(Flag CarBehavior) -> [Flag_BehaviourRecta]
  Longitudinal Dynamics/7(Handling [-] (-inf,inf)) -> [Handling_Recta]
  Longitudinal Dynamics/6(Mass [kg] (0,inf)) -> [Mass_Recta]
  [Bp] -> Longitudinal Dynamics/9(Brake_pedal)
  [Ap] -> Longitudinal Dynamics/8(Gas_pedal)
  [Yaw_error_correction_time] -> Lateral Dynamics/14(Yaw_error_/dt [s])
  In_Numbers/18(Tq_diff_Max [Nm]) -> [Tq_diff_Max]
  In_Numbers/19(Yaw_error_correction_time [s]) -> [Yaw_error_correction_time]
  Sensor_DATA/4(Ellipse_Acc) -> Longitudinal Dynamics/3(Ellipse_Acc), Lateral Dynamics/4(Ellipse_Acc)
  Sensor_DATA/6(GyroEllipse) -> Lateral Dynamics/6(GyroEllipse)
  Gyro_Ellipse/1 -> Sensor_DATA/6(Gyro_Ellipse)
  Ellipse_acc/1 -> Sensor_DATA/4(Ellipse_acc)
  Sensor_DATA/5(YawRate) -> Lateral Dynamics/5(Yaw_Rate)
  [Tq_diff] -> Constraints/21(Tq_diff)
  Wheel_to_engine/1(Tq_diff) -> [Tq_diff]
  Yaw_Rate [rad/s]/1 -> Sensor_DATA/5(Yaw Rate)
  Optimization SKF & CKF/2(CKF_act) -> In_Numbers/2(C-Kamm_Factor), CKF_act/1
  [V_eRL] -> Optimization SKF & CKF/1(RPM_INV1)
  SKF_Initial/1 -> Optimization SKF & CKF/4(SKF_Initial)
  Cte_CKF/1 -> Optimization SKF & CKF/7(Cte_CKF)
  Cte_SKF/1 -> Optimization SKF & CKF/6(Cte_SKF)
  [V_eRR] -> Optimization SKF & CKF/2(RPM_INV2)
  [Steer_An] -> Optimization SKF & CKF/3(Steer_An)
  CKF_Initial/1 -> Optimization SKF & CKF/5(CKF_Initial)
  Optimization SKF & CKF/1(SKF_act) -> In_Numbers/1(S-Kamm_Factor), SKF_act/1
  [Flag_Power] -> Flags/5(Flag_Power)
  [Flag_Temperature] -> Flags/4(Flag_Temperature)
  [Flag_CarBehavior] -> Flags/1(Flag_CarBehavior)
  [Flag_WheelSpin_RR] -> Flags/2(Flag_WheelSpin_RR)
  [Flag_WheelSpin_RL] -> Flags/3(Flag_WheelSpin_RL)
  Flags/1(Flags) -> Flags_[num5]/1
  Constraints/6(Flag_Power) -> [Flag_Power]
  Constraints/5(Flag_Temperature) -> [Flag_Temperature]
  Constant/1 -> MATLAB Function2/1(cte), MATLAB Function1/1(cte)
  MATLAB Function1/1(value) -> [Flag_WheelSpin_RR]
  MATLAB Function2/1(value) -> [Flag_WheelSpin_RL]
  Lateral Dynamics/8(Flag CarBehavior) -> Merge7/2
  Merge7/1 -> [Flag_CarBehavior]
  Limit TemperatureMotor/1 -> In_Numbers/6(Limit Temperature Motor [ºC])
  In_Numbers/14(Temperature limit Motor [ºC]) -> [Temperature_limit_Motor]
  [Temperature_limit_Motor] -> Constraints/12(TemperatureI_limit_Motor)
  [TemperatureMotor] -> Constraints/13(TemperatureIMotor)
  Sensor_DATA/16(TemperatureMotor) -> [TemperatureMotor]
  Sensor_DATA/15(TemperatureIGBT) -> [TemperatureIGBT]
  Temperature Motor [ºC]/1 -> Sensor_DATA/16(Temperature Motor)
  Constraints/4(Tq_RLout) -> Tq_RL [Nm] (0,inf)/1  "Out_RL"
  Constraints/3(Tq_RRout) -> Tq_RR [Nm] (0,inf)/1  "Out_RR"
  [ReductionCte_Temperature] -> Constraints/10(ReductionCte_Temperature)
  Reduction Temperature/1 -> In_Numbers/8(Reduction_T [0-1])
  In_Numbers/16(ReductionCte_Temperature (0-1)) -> [ReductionCte_Temperature]
  Lateral Dynamics/5(Fy_R [N] (0,inf)) -> Merge6/2
  Merge6/1 -> Fy_R [N] (0,inf)/1
  Merge5/1 -> Handling [-] (-inf,inf)/1
  Lateral Dynamics/7(Handling [-] (-inf,inf)) -> Merge5/2
  Lateral Dynamics/6(" Mass [kg] (0,inf)") -> Merge4/2
  Merge4/1 -> Mass [kg] (0,inf)/1
  [ei_Perform] -> Terminator2/1
  [MaxRegTorque] -> Constraints/18(MaxRegTorque)
  Ap_Sat_Down [-]/1 -> In_Numbers/11(Ap_Sat_Down [-])
  Ap_Sat_Up [-]/1 -> In_Numbers/10(Ap_Sat_Up [-])
  Steering Saturation (per site) [deg]/1 -> In_Numbers/9(Steering Saturation (per site) [deg])
  Merge/1 -> Wheel_to_engine/1("Fx_FR ")
  Longitudinal Dynamics/4("Fx_RL ") -> Merge3/1
  Longitudinal Dynamics/3("Fx_RR ") -> Merge2/1
  Longitudinal Dynamics/2(Fx_FL) -> Merge1/1
  Longitudinal Dynamics/1(Fx_FR) -> Merge/1
  [SK_Factor] -> Longitudinal Dynamics/10(SK_Factor)
  [CK_Factor] -> Lateral Dynamics/13(CK_Factor)
  Reduction Power/1 -> In_Numbers/7(Reduction_P [0-1])
  Limit TemperatureIGBT/1 -> In_Numbers/5(Limit TemperatureIGBT [ºC])
  Limit Power [kW]/1 -> In_Numbers/4(Limit Power [kW])
  Max Regen Torque [Nm]/1 -> In_Numbers/3(Max Regen Torque [Nm])
  Merge1/1 -> Wheel_to_engine/2("Fx_FL ")
  Merge2/1 -> Wheel_to_engine/3("Fx_RR "), MaxFx_RR [N] (0,inf)/1
  Merge3/1 -> Wheel_to_engine/4("Fx_RL "), MaxFx_RL [N] (0,inf)/1
  [RT] -> Wheel_to_engine/6(RT)
  [Re] -> Wheel_to_engine/5(Re)
  In_Numbers/4(Cornering Kamm_Factor [0-2]) -> [CK_Factor]
  Constraints/2("Tq_FLout ") -> Terminator1/1
  Constraints/1(Tq_FRout) -> Terminator/1
  Velocity_eRL [rad/s]/1 -> Sensor_DATA/18("V_eRL ")
  Velocity_eRR [rad/s]/1 -> Sensor_DATA/17(V_eRR)
  Temperature IGBTs [ºC]/1 -> Sensor_DATA/15(TemperatureIN)
  Gas Pedal (0-1) [-]/1 -> Sensor_DATA/11(Gas Pedal)
  RL_Susp [N]/1 -> Sensor_DATA/10(RL_Susp)
  F_acc (ax,ay,az) [m/s2]/1 -> Sensor_DATA/2("F_Acc ")
  R_acc (ax,ay,az) [m/s2]/1 -> Sensor_DATA/3(R_Acc)
  FR_Susp [N]/1 -> Sensor_DATA/7(FR_Susp)
  FL_Susp [N]/1 -> Sensor_DATA/8(FL_Susp)
  In_Numbers/13(Temperature limit IGBT [ºC]) -> [Temperature_limit_IGBT]
  [V_eRL] -> Constraints/16(V_eRL)
  Brake Pedal (0-1) [-]/1 -> Sensor_DATA/12(Brake Pedal)
  Regenerative Enable [0,1]/1 -> Sensor_DATA/13(Regenerative Enable)
  [V_eRR] -> Constraints/15(V_eRR)
  Sensor_DATA/17("V_eRR ") -> [V_eRR]
  Sensor_DATA/14(Power) -> [Power]
  Power [kW]/1 -> Sensor_DATA/14("Power ")
  RR_Susp [N]/1 -> Sensor_DATA/9(RR_Susp)
  [Tq_max] -> Constraints/17(Tq_max)
  [Bp] -> Driver / CarBehaviours/5(Bp)  "Bp"
  In_Numbers/9(Engine+Inverter Performance[-]) -> [ei_Perform]
  [Reg_enable] -> Constraints/20(Reg_enable)
  [TemperatureIGBT] -> Constraints/11(TemperatureIGBT)
  In_Numbers/17(MaxRegTorque [Nm]) -> [MaxRegTorque]
  Sensor_DATA/18(V_eRL) -> [V_eRL]
  [Bp] -> Constraints/19(Bp)
  [Temperature_limit_IGBT] -> Constraints/14(Temperature_limit_IGBT)
  [Trans_max_static] -> Constraints/5("Trans_max_static ")
  Driver / CarBehaviours/1(Tq_FRout) -> Constraints/1(Tq_FRin)
  Wheel_to_engine/2(Tq_FR) -> Driver / CarBehaviours/1(Tq_FRin)
  Steering_Angle [deg]/1 -> Sensor_DATA/1(Steer_Ang), [Steer_An]
  Driver / CarBehaviours/2("Tq_FLout ") -> Constraints/2(Tq_FLin)
  Driver / CarBehaviours/4(Tq_RLout) -> Constraints/4("Tq_RL_wc "), Tq_RLwc [Nm] (0,inf)/1  "Teo_RL"
  [Ap_Sat_down] -> Driver / CarBehaviours/9(Ap_Sat_down)
  In_Numbers/12("Power limit [KW] ") -> [Power_limit]
  [Power] -> Constraints/7(Power)
  [Ap] -> Driver / CarBehaviours/6(Ap)  "Ap"
  In_Numbers/10(Trans_max _static[Nm]) -> [Trans_max_static]
  [Ap_Sat_up] -> Driver / CarBehaviours/8(Ap_Sat_up)
  [ReductionCte_Power] -> Constraints/9(ReductionCte_Power)
  [Reg_enable] -> Driver / CarBehaviours/7(Reg_enable)
  In_Numbers/11(Trans_max_dynamic [Nm]) -> [Trans_max_dynamic]
  Wheel_to_engine/3(Tq_FL) -> Driver / CarBehaviours/2(Tq_FLin)
  Wheel_to_engine/4(Tq_RR) -> MATLAB Function2/2(v), MaxTq_RR [Nm] (0,inf)/1, Driver / CarBehaviours/3(Tq_RRin)  "Tq_RR"
  Driver / CarBehaviours/5(out_Throttle) -> Throttle [0-1] (0-100%)/1  "Out"
  In_Numbers/15(ReductionCte_Power (0-1)) -> [ReductionCte_Power]
  [Power_limit] -> Constraints/8(Power_limit)
  [Trans_max_dynamic] -> Constraints/6(Trans_max_dynamic)
  Wheel_to_engine/5(Tq_RL) -> MATLAB Function1/2(v), MaxTq_RL [Nm] (0,inf)/1, Driver / CarBehaviours/4("Tq_RLin ")  "Tq_RL"
  Sensor_DATA/1(Steer_ang) -> Lateral Dynamics/1(Steering_Angle), "Steer_ang is in Steer_Sat range ---> Long Steer_ang is not in Steer_Sat range -> Lat "/2
  Sensor_DATA/7(FR_susp) -> Longitudinal Dynamics/4(FR_susp), Lateral Dynamics/7(FR_susp)
  Sensor_DATA/13(Reg_Enable) -> [Reg_enable]
  Sensor_DATA/8(FL_susp) -> Longitudinal Dynamics/5(FL_susp), Lateral Dynamics/8(FL_susp)
  Sensor_DATA/12(Brake_Pedal) -> Lateral Dynamics/12(Brake_pedal), [Bp]
  Sensor_DATA/3(R_acc) -> Longitudinal Dynamics/2(R_acc), Lateral Dynamics/3(R_acc)
  Sensor_DATA/2(F_acc) -> Longitudinal Dynamics/1(F_acc), Lateral Dynamics/2(F_acc)
  Driver / CarBehaviours/3(Tq_RRout) -> Constraints/3(Tq_RR_wc), Tq_RRwc [Nm] (0,inf)/1  "Teo_RR"
  In_Numbers/7(Ap_Sat_down[-]) -> [Ap_Sat_down]
  In_Numbers/8(Ap_Sat_up[-]) -> [Ap_Sat_up]
  Sensor_DATA/9(RR_susp) -> Longitudinal Dynamics/6(RR_susp), Lateral Dynamics/9(RR_susp)
  In_Numbers/5(Transmision_Ratio[-]) -> [RT]
  In_Numbers/6(Effective Rolling Radius[m]) -> [Re]
  Sensor_DATA/11(Gas_Pedal) -> Lateral Dynamics/11(Gas_pedal), [Ap]
  In_Numbers/2(Tq_Max [Nm]) -> [Tq_max]
  In_Numbers/1(Steer_Sat [deg]) -> "Steer_ang is in Steer_Sat range ---> Long Steer_ang is not in Steer_Sat range -> Lat "/1
  In_Numbers/3(Straight Kamm_Factor [0-2]) -> [SK_Factor]
  Sensor_DATA/10(RL_susp) -> Longitudinal Dynamics/7(RL_susp), Lateral Dynamics/10(RL_susp)
  "Steer_ang is in Steer_Sat range ---> Long Steer_ang is not in Steer_Sat range -> Lat "/2 -> Lateral Dynamics/Action
  "Steer_ang is in Steer_Sat range ---> Long Steer_ang is not in Steer_Sat range -> Lat "/1 -> Longitudinal Dynamics/Action

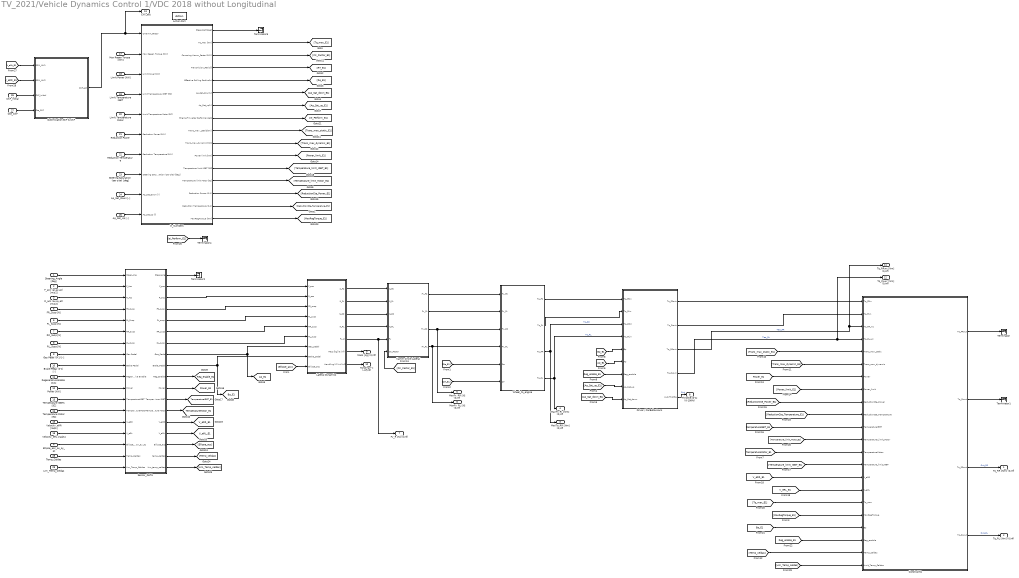
== system TV_2021/Vehicle Dynamics Control 1/VDC 2018 without Longitudinal ==
  Steering_Angle [deg] : Inport
  F_acc (ax,ay,az) [m/s2] : Inport  Port=2
  R_acc (ax,ay,az) [m/s2] : Inport  Port=3
  Ellipse_acc_ax_ay_az : Inport  Port=4
  FR_Susp [N] : Inport  Port=5
  FL_Susp [N] : Inport  Port=6
  RR_Susp [N] : Inport  Port=7
  RL_Susp [N] : Inport  Port=8
  Gas Pedal (0-1) [-] : Inport  Port=9
  Brake Pedal (0-1) [-] : Inport  Port=10
  Regenerative Enable [0,1] : Inport  Port=11
  Power [kW] : Inport  Port=12
  Temperature IGBTs [ºC] : Inport  Port=13
  Temperature Motor [ºC] : Inport  Port=14
  Velocity_eRR [rad/s] : Inport  Port=15
  Velocity_eRL [rad/s] : Inport  Port=16
  Max Regen Torque [Nm] : Inport  Port=17
  Limit Power [kW] : Inport  Port=18
  Limit Temperature IGBT : Inport  Port=19
  Limit Temperature Motor : Inport  Port=20
  Reduction Power : Inport  Port=21
  Reduction Temperature : Inport  Port=22
  Steering Saturation (per site) [deg] : Inport  Port=23
  Ap_Sat_Down [-] : Inport  Port=24
  Ap_Sat_Up [-] : Inport  Port=25
  CKF_Initial : Inport  Port=26
  Cte_CKF : Inport  Port=27
  Temp_Celdas : Inport  Port=28
  Lim_Temp_Celdas : Inport  Port=29
  Action Port : ActionPort
  Constraints : Subsystem
  Driver / CarBehaviours : Subsystem
  In_Numbers : Subsystem
  Kamm Circle Lateral : Subsystem
  Lateral Dynamics : Subsystem
  Optimization SKF & CKF : Subsystem
  Sensor_DATA : Subsystem
  Terminator{,1..2,4..5} (5 alike) : Terminator
  Wheel_to_engine : Subsystem
  Tq_RR [Nm] (0,inf) : Outport
  Tq_RL [Nm] (0,inf) : Outport  Port=2
  MaxTq_RR [Nm] (0,inf) : Outport  Port=3
  MaxTq_RL [Nm] (0,inf) : Outport  Port=4
  MaxFx_RR [N] (0,inf) : Outport  Port=5
  MaxFx_RL [N] (0,inf) : Outport  Port=6
  Fy_R [N] (0,inf) : Outport  Port=7
  Throttle [0-1] (0-100%) : Outport  Port=8
  Mass [kg] (0,inf) : Outport  Port=9
  Handling [-] (-inf,inf) : Outport  Port=10
  Tq_RRwc [Nm] (0,inf) : Outport  Port=11
  Tq_RLwc [Nm] (0,inf) : Outport  Port=12
  CKF_act : Outport  Port=13
  tag scope: Ap_E1=global, Bp_E1=global, Power_E1=global, Reg_enable_E1=global, TemperatureIGBT_E1=global, TemperatureMotor_E1=global, V_eRL_E1=global, V_eRR_E1=global
  wires:
  [Lim_Temp_celdas] -> Constraints/22(Limit_Temp_Celdas)
  [Temp_celdas] -> Constraints/21(Temp_celdas)
  Sensor_DATA/18(Lim_temp_celdas) -> [Lim_Temp_celdas]
  Sensor_DATA/17(temp_celdas) -> [Temp_celdas]
  Lim_Temp_Celdas/1 -> Sensor_DATA/18(Lim_Temp_Celdas)
  Temp_Celdas/1 -> Sensor_DATA/17(Temp_Celdas)
  [Ellipse_acc] -> Lateral Dynamics/9(Ellipse_acc)
  Lateral Dynamics/5(Fy_R) -> Fy_R [N] (0,inf)/1, Kamm Circle Lateral/5(Fy)
  Sensor_DATA/16(Ellipse_acc) -> [Ellipse_acc]
  Ellipse_acc_ax_ay_az/1 -> Sensor_DATA/16(Ellipse_acc_ax_ay_az)
  Constraints/4(Tq_RLout) -> Tq_RL [Nm] (0,inf)/1  "Out_RL"
  Constraints/3(Tq_RRout) -> Tq_RR [Nm] (0,inf)/1  "Out_RR"
  [V_eRL_E1] -> Optimization SKF & CKF/1(RPM_INV1)
  Optimization SKF & CKF/1(CKF_act) -> In_Numbers/1(C-Kamm_Factor), CKF_act/1
  Cte_CKF/1 -> Optimization SKF & CKF/4(Cte_CKF)
  CKF_Initial/1 -> Optimization SKF & CKF/3(CKF_Initial)
  [V_eRR_E1] -> Optimization SKF & CKF/2(RPM_INV2)
  Sensor_DATA/13(Temperature Motor) -> [TemperatureMotor_E1]
  Temperature Motor [ºC]/1 -> Sensor_DATA/13(TemperatureMotor)
  In_Numbers/13(Temperature limit Motor [ºC]) -> [Temperature_limit_Motor_E1]
  Limit Temperature Motor/1 -> In_Numbers/5(Limit Temperature Motor [ºC])
  [Temperature_limit_Motor_E1] -> Constraints/12(TemperatureI_limit_Motor)
  [TemperatureMotor_E1] -> Constraints/13(TemperatureIMotor)
  [ReductionCte_Temperature_E1] -> Constraints/10(ReductionCte_Temperature)
  [MaxRegTorque_E1] -> Constraints/18(MaxRegTorque)
  Constraints/2("Tq_FLout ") -> Terminator1/1
  Constraints/1(Tq_FRout) -> Terminator/1
  [V_eRL_E1] -> Constraints/16(V_eRL)
  [V_eRR_E1] -> Constraints/15(V_eRR)
  [Tq_max_E1] -> Constraints/17(Tq_max)
  [Reg_enable_E1] -> Constraints/20(Reg_enable)
  [TemperatureIGBT_E1] -> Constraints/11(TemperatureIGBT)
  [Bp_E1] -> Constraints/19(Bp)
  [Temperature_limit_IGBT_E1] -> Constraints/14(Temperature_limit_IGBT)
  [Trans_max_static_E1] -> Constraints/5("Trans_max_static ")
  Driver / CarBehaviours/1(Tq_FRout) -> Constraints/1(Tq_FRin)
  Driver / CarBehaviours/2("Tq_FLout ") -> Constraints/2(Tq_FLin)
  Driver / CarBehaviours/4(Tq_RLout) -> Constraints/4("Tq_RL_wc "), Tq_RLwc [Nm] (0,inf)/1  "Teo_RL"
  [Power_E1] -> Constraints/7(Power)
  [ReductionCte_Power_E1] -> Constraints/9(ReductionCte_Power)
  [Power_limit_E1] -> Constraints/8(Power_limit)
  [Trans_max_dynamic_E1] -> Constraints/6(Trans_max_dynamic)
  Driver / CarBehaviours/3(Tq_RRout) -> Constraints/3(Tq_RR_wc), Tq_RRwc [Nm] (0,inf)/1  "Teo_RR"
  Reduction Temperature/1 -> In_Numbers/7(Reduction Temperature [0-1])
  In_Numbers/15(Reduction Temperature (0-1)) -> [ReductionCte_Temperature_E1]
  Lateral Dynamics/7(Handling [-] (-inf,inf)) -> Handling [-] (-inf,inf)/1
  Lateral Dynamics/6(Mass [kg] (0,inf)) -> Mass [kg] (0,inf)/1
  In_Numbers/1(Steer_Sat [deg]) -> Terminator5/1
  [ei_Perform_E1] -> Terminator4/1
  Driver / CarBehaviours/5(out_Throttle) -> Throttle [0-1] (0-100%)/1  "Out"
  Lateral Dynamics/4(N_RL) -> Kamm Circle Lateral/4(N_RL)
  Lateral Dynamics/3("N_RR ") -> Kamm Circle Lateral/3(N_RR)
  Lateral Dynamics/2("N_FL ") -> Kamm Circle Lateral/2(N_FL)
  Lateral Dynamics/1(N_FR) -> Kamm Circle Lateral/1("N_FR ")
  Sensor_DATA/1(Steer_ang) -> Terminator2/1
  Kamm Circle Lateral/4("Fx_RL ") -> Wheel_to_engine/4("Fx_RL "), MaxFx_RL [N] (0,inf)/1
  Kamm Circle Lateral/3("Fx_RR ") -> Wheel_to_engine/3("Fx_RR "), MaxFx_RR [N] (0,inf)/1
  Kamm Circle Lateral/2(Fx_FL) -> Wheel_to_engine/2("Fx_FL ")
  Kamm Circle Lateral/1(Fx_FR) -> Wheel_to_engine/1("Fx_FR ")
  [CK_Factor_E1] -> Kamm Circle Lateral/6(CK_Factor)
  Steering Saturation (per site) [deg]/1 -> In_Numbers/8(Steering Saturation (per site) [deg])
  Ap_Sat_Down [-]/1 -> In_Numbers/9(Ap_Sat_Down [-])
  Ap_Sat_Up [-]/1 -> In_Numbers/10(Ap_Sat_Up [-])
  [RT_E1] -> Wheel_to_engine/6(RT)
  [Re_E1] -> Wheel_to_engine/5(Re)
  In_Numbers/3(Cornering Kamm_Factor [0-2]) -> [CK_Factor_E1]
  Reduction Power/1 -> In_Numbers/6(Reduction Power [0-1])
  Limit Temperature IGBT/1 -> In_Numbers/4(Limit Temperature IGBT [ºC])
  Limit Power [kW]/1 -> In_Numbers/3(Limit Power [kW])
  Max Regen Torque [Nm]/1 -> In_Numbers/2(Max Regen Torque [Nm])
  Velocity_eRL [rad/s]/1 -> Sensor_DATA/15("V_eRL ")
  Velocity_eRR [rad/s]/1 -> Sensor_DATA/14(V_eRR)
  Temperature IGBTs [ºC]/1 -> Sensor_DATA/12(TemperatureIGBT)
  Gas Pedal (0-1) [-]/1 -> Sensor_DATA/8(Gas Pedal)
  RL_Susp [N]/1 -> Sensor_DATA/7(RL_Susp)
  F_acc (ax,ay,az) [m/s2]/1 -> Sensor_DATA/2("F_Acc ")
  R_acc (ax,ay,az) [m/s2]/1 -> Sensor_DATA/3(R_Acc)
  FR_Susp [N]/1 -> Sensor_DATA/4(FR_Susp)
  FL_Susp [N]/1 -> Sensor_DATA/5(FL_Susp)
  In_Numbers/12(Temperature limit IGBT [ºC]) -> [Temperature_limit_IGBT_E1]
  Brake Pedal (0-1) [-]/1 -> Sensor_DATA/9(Brake Pedal)
  Regenerative Enable [0,1]/1 -> Sensor_DATA/10(Regenerative Enable)
  Sensor_DATA/14("V_eRR ") -> [V_eRR_E1]
  Sensor_DATA/11(Power) -> [Power_E1]
  Power [kW]/1 -> Sensor_DATA/11("Power ")
  RR_Susp [N]/1 -> Sensor_DATA/6(RR_Susp)
  Sensor_DATA/12(Temperature IGBT) -> [TemperatureIGBT_E1]
  [Bp_E1] -> Driver / CarBehaviours/5(Bp)
  In_Numbers/8(Engine+Inverter Performance[-]) -> [ei_Perform_E1]
  In_Numbers/16(MaxRegTorque [Nm]) -> [MaxRegTorque_E1]
  Sensor_DATA/15(V_eRL) -> [V_eRL_E1]
  Wheel_to_engine/1(Tq_FR) -> Driver / CarBehaviours/1(Tq_FRin)
  Steering_Angle [deg]/1 -> Sensor_DATA/1(Steer_Ang)
  [Ap_Sat_down_E1] -> Driver / CarBehaviours/9(Ap_Sat_down)
  In_Numbers/11("Power limit [KW] ") -> [Power_limit_E1]
  [Ap_E1] -> Driver / CarBehaviours/6(Ap)
  In_Numbers/9(Trans_max _static[Nm]) -> [Trans_max_static_E1]
  [Ap_Sat_up_E1] -> Driver / CarBehaviours/8(Ap_Sat_up)
  [Reg_enable_E1] -> Driver / CarBehaviours/7(Reg_enable)
  In_Numbers/10(Trans_max_dynamic [Nm]) -> [Trans_max_dynamic_E1]
  Wheel_to_engine/2(Tq_FL) -> Driver / CarBehaviours/2(Tq_FLin)
  Wheel_to_engine/3(Tq_RR) -> MaxTq_RR [Nm] (0,inf)/1, Driver / CarBehaviours/3(Tq_RRin)  "Tq_RR"
  In_Numbers/14(Reduction Power (0-1)) -> [ReductionCte_Power_E1]
  Wheel_to_engine/4(Tq_RL) -> MaxTq_RL [Nm] (0,inf)/1, Driver / CarBehaviours/4("Tq_RLin ")  "Tq_RL"
  Sensor_DATA/4(FR_susp) -> Lateral Dynamics/3(FR_susp)
  Sensor_DATA/10(Reg_Enable) -> [Reg_enable_E1]
  Sensor_DATA/5(FL_susp) -> Lateral Dynamics/4(FL_susp)
  Sensor_DATA/9(Brake_Pedal) -> Lateral Dynamics/8(Brake_pedal), [Bp_E1]
  Sensor_DATA/3(R_acc) -> Lateral Dynamics/2(R_acc)
  Sensor_DATA/2(F_acc) -> Lateral Dynamics/1(F_acc)
  In_Numbers/6(Ap_Sat_down[-]) -> [Ap_Sat_down_E1]
  In_Numbers/7(Ap_Sat_up[-]) -> [Ap_Sat_up_E1]
  Sensor_DATA/6(RR_susp) -> Lateral Dynamics/5(RR_susp)
  In_Numbers/4(Transmision_Ratio[-]) -> [RT_E1]
  In_Numbers/5(Effective Rolling Radius[m]) -> [Re_E1]
  Sensor_DATA/8(Gas_Pedal) -> Lateral Dynamics/7(Gas_pedal), [Ap_E1]
  In_Numbers/2(Tq_Max [Nm]) -> [Tq_max_E1]
  Sensor_DATA/7(RL_susp) -> Lateral Dynamics/6(RL_susp)

== system TV_2021/Vehicle Dynamics Control 2018/Rigid Axle ==
  "Ap_Sat_up " : Inport
  Ap_Sat_down : Inport  Port=2
  Gas Pedal [0-1] : Inport  Port=3
  Action Port : ActionPort
  Accelerating : Subsystem
  Torque_RL [Nm] : Constant  Value=60
  Torque_RR [Nm] : Constant  Value=60
  Tq_RR_E3 : Outport
  Tq_RL_E3 : Outport  Port=2
  wires:
  Torque_RR [Nm]/1 -> Accelerating/4(Tq_RR)
  Torque_RL [Nm]/1 -> Accelerating/5("Tq_RL ")
  Accelerating/2(Tq_RL) -> Tq_RL_E3/1
  Accelerating/1("Tq_RR ") -> Tq_RR_E3/1
  Gas Pedal [0-1]/1 -> Accelerating/1(Ap)
  "Ap_Sat_up "/1 -> Accelerating/2("Ap_Sat_up ")
  Ap_Sat_down/1 -> Accelerating/3(Ap_Sat_down)
